simulink model "motor_model"  (R2025b)
settings: Solver=FixedStepAuto  StartTime=0.0  StopTime=10.0  FixedStep=0.25e-3  RelTol=1e-3
values from neighbouring files (symbols this model uses):
  B = 0    [params_motor.m]    (also in plot_basic_vi_log.m)
  J = 115*1e-7    (= 1.15e-05)    [params_motor.m]    (also in plot_basic_vi_log.m)
  Ke = Kt    (= 0.0797)    [params_motor.m]    (also in plot_basic_vi_log.m)
  Kt = 79.7e-3    (= 0.0797)    [params_motor.m]    (also in plot_basic_vi_log.m)
  L = 708e-6    (= 0.000708)    [params_motor.m]    (also in plot_basic_vi_log.m)
  Mr = 6.5e-3    (= 0.0065)    [params_motor.m]    (also in plot_basic_vi_log.m)
  R = 2.59    [params_motor.m]    (also in plot_basic_vi_log.m)
settings Model: Creator=farfar  LastModifiedBy=farfar

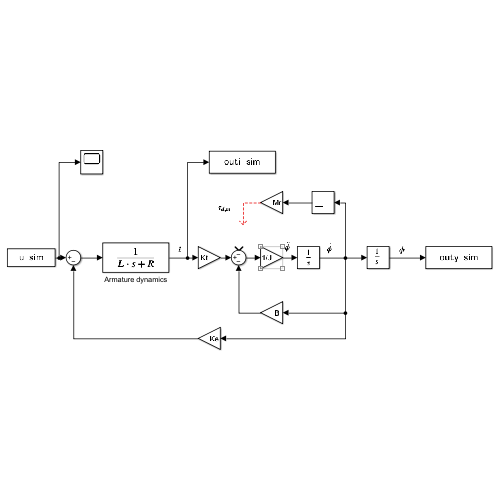
[thumbnail: Simulink's stored preview of the top-level diagram]
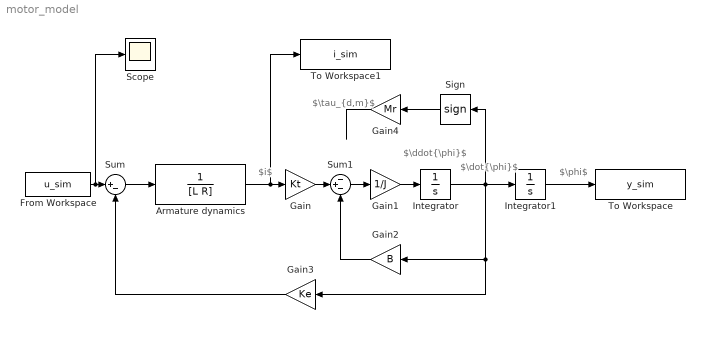
== system motor_model ==
  note: $\phi$
  note: $i$
  note: $\ddot{\phi}$
  note: $\tau_{d,m}$
  note: $\dot{\phi}$
  Armature dynamics : TransferFcn  Denominator=[L R]
  From Workspace : FromWorkspace  VariableName=u_sim
  Gain : Gain  Gain=Kt
  Gain1 : Gain  Gain=1/J
  Gain2 : Gain  Gain=B
  Gain3 : Gain  Gain=Ke
  Gain4 : Gain  Gain=Mr
  Integrator : Integrator
  Integrator1 : Integrator
  Scope : Scope
      settings: ActiveDisplayYMinimum=-1  ActiveDisplayYMaximum=1
  Sign : Signum  ZeroCross=off
  Sum : Sum  Inputs=|+-
  Sum1 : Sum  Inputs=-+-
  To Workspace : ToWorkspace  VariableName=y_sim  SampleTime=5e-3
  To Workspace1 : ToWorkspace  VariableName=i_sim  SampleTime=5e-3
  wires:
  Armature dynamics/1 -> To Workspace1/1, Gain/1
  Gain/1 -> Sum1/2
  Sum1/1 -> Gain1/1
  Gain1/1 -> Integrator/1
  Sign/1 -> Gain4/1
  Gain2/1 -> Sum1/3
  Integrator/1 -> Gain3/1, Gain2/1, Integrator1/1, Sign/1
  Sum/1 -> Armature dynamics/1
  Gain3/1 -> Sum/2
  Integrator1/1 -> To Workspace/1
  From Workspace/1 -> Scope/1, Sum/1
  Gain4/1 -> ?
